simulink model "modele5Bhrolv2"  (R2024a)
settings: Solver=VariableStepAuto  StartTime=0.0  StopTime=100  RelTol=10e-2
undefined symbols (not defined in the file or in its folder): A_L, A_S, C_x, calcul_adherence, calcul_delta, calcul_forceaero, calcul_forces, calcul_lambda, calcul_moteur, calcul_N, calcul_omega, calcul_omegaackermann, calcul_retourvitesse, calcul_rotaroute, calcul_slipangle, calcul_vitessesroues, check_zeros_1, check_zeros_8, Cte_1, Cte_2, Cte_3, Cte_4, d_f, d_r, EPSILON, eqpfd, f, g, h, Iz, J, L, l_f, l_r, M, projection, R, reconstructionPi, rho
libraries: simulink x5, embmathops x1, slpidlib x1
settings Model: Creator=TP-EEA  LastModifiedBy=TP-EEA

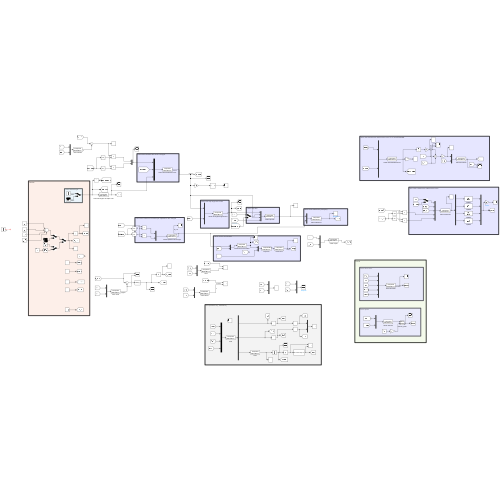
[thumbnail: Simulink's stored preview of the top-level diagram]
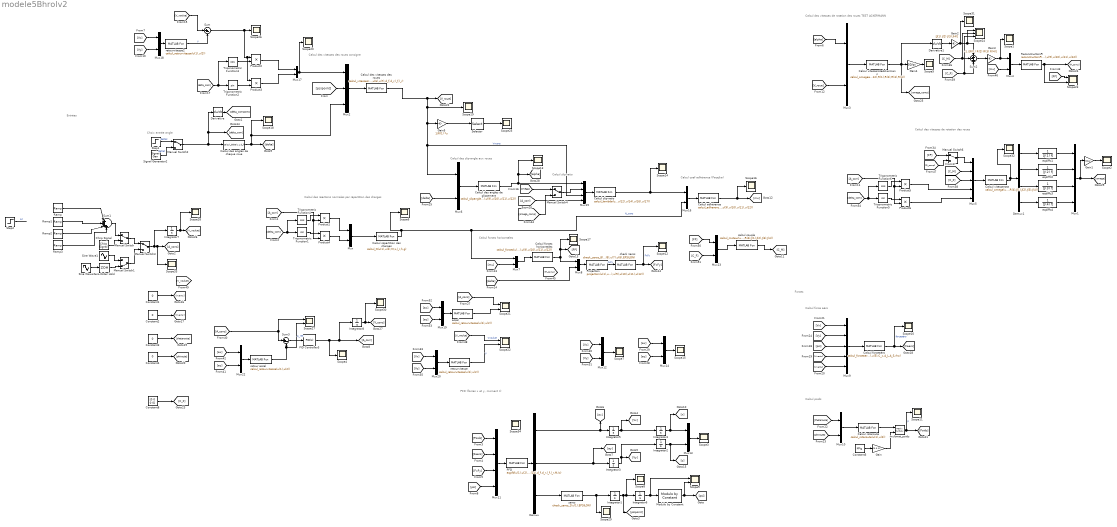
== system modele5Bhrolv2 ==
  note: Calcul des vitesses des roues consigne
  note: Entrées
  note: Choix entrée angle
  note: Calcul des vitesses de rotation des roues
  note: PFD (forces x et y, moment z)
  note: Calcul poids
  note: Calcul des slip-angle aux roues
  note: Calcul coef adhérence (Pacejka)
  note: Calcul slip-ratio
  note: Calcul des réactions normales par répartition des charges
  note: Calcul forces horizontales
  note: Forces
  note: Calcul force aéro
  note: Calcul des vitesses de rotation des roues TEST ACKERMANN
  Calcul adhérence : MATLABFcn  MATLABFcn=calcul_adherence(u(1),u(2),u(3),u(4),u(5),u(6),u(7),u(8),Cte_1,Cte_2,Cte_3,Cte_4,u(9),u(10),u(11),u(12))  OutputDimensions=4*2
  Calcul des angles de chaque roue : MATLABFcn  MATLABFcn=calcul_delta(u,L,d_f)  OutputDimensions=4
  Calcul des angles de glissement : MATLABFcn  MATLABFcn=calcul_slipangle(u(1),u(2),u(3),u(4),u(5),u(6),u(7),u(8),u(9),u(10),u(11),u(12))  OutputDimensions=4
  Calcul des vitesses des roues : MATLABFcn  MATLABFcn=calcul_vitessesroues(u(1),u(2),u(3),u(4),u(5),u(6),u(7),d_f,d_r,l_f,l_r)  OutputDimensions=8
  Calcul forceaéro : MATLABFcn  MATLABFcn=calcul_forceaero(u(1),u(2),u(3),u(4),u(5),C_x,A_L,A_S,rho)  OutputDimensions=2
  Calcul forces horizontales : MATLABFcn  MATLABFcn=calcul_forces(u(1),u(2),u(3),u(4),u(5),u(6),u(7),u(8),u(9),u(10),u(11),u(12))  OutputDimensions=4*2
  Calcul rotaroute : MATLABFcn  MATLABFcn=calcul_rotaroute(u(1),u(2))  OutputDimensions=[3 3]  Output1D=off
  Calcul répartition des charges : MATLABFcn  MATLABFcn=calcul_N(u(1),u(2),M,L,l_r,h,g)  OutputDimensions=4
  Calcul slip-ratio : MATLABFcn  MATLABFcn=calcul_lambda(u(1),u(2),u(3),u(4),R(1),R(2),R(3),R(4),u(5),u(6),u(7),u(8),u(9),u(11),u(13),u(15),u(10),u(12),u(14),u(16),u(17))  OutputDimensions=4*2
  Calcul vitesserota : MATLABFcn  MATLABFcn=calcul_omega(u(1),u(2),u(3),u(4),u(5),u(6),u(7),u(8),u(9),u(10),u(11),u(12),u(13),u(14),u(15),u(16),u(17),u(18),R(1),R(2),R(3),R(4),J(1),J(2),J(3),J(4))  OutputDimensions=4
  Calcul vitesserotaAckermann : MATLABFcn  MATLABFcn=calcul_omegaackermann(u(1),u(2),u(3),u(4),u(5),u(6),u(7),u(8),u(9),u(10),u(11),u(12),R(1),R(2),R(3),R(4))  OutputDimensions=4
  Chirp Signal : simulink/Sources/Chirp Signal  f1=0.1  T=100  f2=1
  Constant{1..4} (4 alike) : Constant  Value=0
  Constant5 : Constant  Value=M*g  VectorParams1D=off
  Constant8 : Constant  Value=[0 0 0 0]
  Demux : Demux  Outputs=3
  Demux1 : Demux
  Derivative : Derivative
  Derivative1 : Derivative
  Gain : Gain  Gain=[0 0 1]'
  Gain1 : Gain  Gain=30/pi
  Gain2 : Gain  Gain=[J(1) J(2) J(3) J(4)]
  Gain3 : Gain  Gain=-1./[R(1) R(2) R(3) R(4)]
  Gain4 : Gain  Gain=30/pi
  Gain5 : Gain  Gain=1/R(1)  Multiplication=Matrix(K*u)
  Integrator{1..8} (8 alike) : Integrator
  Manual Switch{,2..4,6} (5 alike) : ManualSwitch
  Manual Switch1 : ManualSwitch  CurrentSetting=0
  Modulo by Constant : embmathops/Modulo by Constant  Denominator=2*pi  SimulateUsing=Code generation
      settings: LibrarySourceBlock=embeddedMathLib/Modulo by Constant
  Mux{,3..4,6..8,10,12..14,16..20,22..23} (17 alike) : Mux  Inputs=2
  Mux1 : Mux
  Mux11 : Mux
  Mux15 : Mux
  Mux2 : Mux  Inputs=3
  Mux5 : Mux  Inputs=5
  Mux9 : Mux  Inputs=5
  PFD : MATLABFcn  MATLABFcn=eqpfd(u(1),u(2),u(4),u(5),u(6),u(7),u(8),u(9),u(10),u(11),u(12),u(13),u(14),d_f,d_r,l_f,l_r,M,Iz)  OutputDimensions=3
  PID Controller3 : slpidlib/PID Controller  Controller=PID  Form=Ideal  TimeDomain=Continuous-time  UseExternalTs=off  SampleTime=-1  IntegratorMethod=Forward Euler  FilterMethod=Forward Euler  ControllerParametersSource=internal  P=1  I=30  UseKiTs=off  D=0  UseExternalDerivativeSource=off  N=300  UseFilter=on  TunerSelectOption=Frequency Response Based  InitialConditionSource=internal  InitialConditionForIntegrator=0  InitialConditionForFilter=0  DifferentiatorICPrevScaledInput=0  ExternalReset=none  TrackingMode=off  Kt=1  LimitOutput=off  SatLimitsSource=internal  UpperSaturationLimit=inf  LowerSaturationLimit=-inf  LinearizeAsGain=on  AntiWindupMode=none  Kb=1  LimitIntegrator=off  UpperIntegratorSaturationLimit=inf  LowerIntegratorSaturationLimit=-inf  POutMin=[]  POutMax=[]  IOutMin=[]  IOutMax=[]  DOutMin=[]  DOutMax=[]  NOutMin=[]  NOutMax=[]  SumOutMin=[]  SumOutMax=[]  SaturationOutMin=[]  SaturationOutMax=[]  PParamMin=[]  PParamMax=[]  IParamMin=[]  IParamMax=[]  DParamMin=[]  DParamMax=[]  NParamMin=[]  NParamMax=[]  KbParamMin=[]  KbParamMax=[]  KtParamMin=[]  KtParamMax=[]  KbOutMin=[]  KbOutMax=[]  KtOutMin=[]  KtOutMax=[]  IntegratorOutMin=[]  IntegratorOutMax=[]  FilterOutMin=[]  FilterOutMax=[]  SumI1OutMin=[]  SumI1OutMax=[]  SumI2OutMin=[]  SumI2OutMax=[]  SumI3OutMin=[]  SumI3OutMax=[]  SumI4OutMin=[]  SumI4OutMax=[]  SumDOutMin=[]  SumDOutMax=[]  DifferentiatorOutMin=[]  DifferentiatorOutMax=[]  FilterDiffOutCoefMin=[]  FilterDiffOutCoefMax=[]  ReciprocalOutMin=[]  ReciprocalOutMax=[]  SumDenOutMin=[]  SumDenOutMax=[]  SumNumOutMin=[]  SumNumOutMax=[]  DivideOutMin=[]  DivideOutMax=[]  UdiffTsProdOutMin=[]  UdiffTsProdOutMax=[]  NTsProdOutMin=[]  NTsProdOutMax=[]  UintegralTsProdOutMin=[]  UintegralTsProdOutMax=[]  UngainTsProdOutMin=[]  UngainTsProdOutMax=[]  ClampingZeroOutDataTypeStr=Inherit: Inherit via back propagation  ClampingZeroOutMin=[]  ClampingZeroOutMax=[]  FilterDenConstantOutDataTypeStr=Inherit: Inherit via back propagation  FilterDenConstantOutMin=[]  FilterDenConstantOutMax=[]  PCopyOutDataTypeStr=Inherit: Inherit via back propagation  PCopyOutMin=[]  PCopyOutMax=[]  NCopyOutDataTypeStr=Inherit: Inherit via back propagation  NCopyOutMin=[]  NCopyOutMax=[]  IntegratorContinuousStateAttributes=''  IntegratorStateMustResolveToSignalObject=off  IntegratorRTWStateStorageClass=Auto  FilterContinuousStateAttributes=''  FilterStateMustResolveToSignalObject=off  FilterRTWStateStorageClass=Auto  ParallelPVariant=Passthrough  IdealPVariant=InternalParameters  IVariant=InternalParameters  DVariant=InternalParameters  IntegratorVariant=Continuous  SatVariant=Disabled  AWVariant=Passthrough  PCopyVariant=Disabled  TRVariant=Disabled  FdbkBlocksVariant=Forward  IdealPFdbkVariant=Disabled  SatFdbkVariant=Disabled  DerivativeFilterVariant=ContFilter  NVariant=InternalParameters  NCopyVariant=Disabled  FilterICVariant=InternalICsFilter  IntegratorICVariant=InternalICs  ExternalResetVariant=Disabled  TRSumVariant=Passthrough  SumFdbkVariant=Disabled  SumVariant=Sum_PID  TsampFilterVariant=InternalTs  TsampNgainVariant=Passthrough  TsampIntegralVariant=Disabled_SignalSpec  ExternalSaturationOutDataTypeStr=Inherit: Same as second input  DerivativeSourceVariant=ErrorSignal
  Product{1..6} (6 alike) : Product
  Projection : MATLABFcn  MATLABFcn=projection(u(1),u(2),u(3),u(4),u(5),u(6),u(7),u(8),u(9),u(10),u(11),u(12))  OutputDimensions=8
  Ramp : simulink/Sources/Ramp  slope=1  start=0  InitialOutput=0
  Ramp1 : simulink/Sources/Ramp  slope=-1  start=3  InitialOutput=0
  Ramp2 : simulink/Sources/Ramp  slope=-1  start=7  InitialOutput=0
  Ramp3 : simulink/Sources/Ramp  slope=1  start=9  InitialOutput=0
  ReconstructionPi : MATLABFcn  MATLABFcn=reconstructionPi(u(1),u(2),u(3),u(4),u(5),u(6),u(7),u(8),u(9),u(10),u(11),u(12))  OutputDimensions=8
  Scope{1..8,10..20,25..26,28..34} (28 alike) : Scope
  Scope{9,21..23,27} (5 alike) : Scope  NumInputPorts=2
  Scope24 : Scope  NumInputPorts=3
  Selector : Selector  InputPortWidth=8  IndexOptions=Index vector (dialog)  Indices=[1,3,5,7]  OutputSizes=1
  Signal Generator2 : SignalGenerator  Frequency=0.01  Units=rad/sec
  Sine Wave : Sin  SampleTime=0
  Sine Wave1 : Sin  SampleTime=0
  Step1 : Step  Time=0  After=0  SampleTime=0
  Step2 : Step  Time=3  After=3  SampleTime=0
  Sum : Sum  Inputs=|+-
  Sum1 : Sum  Inputs=|++++
  Sum2 : Sum  Inputs=+-+
  Sum3 : Sum  Inputs=|+-
  Trigonometric Function1 : Trigonometry
  Trigonometric Function2 : Trigonometry
  Trigonometric Function3 : Trigonometry  Operator=cos
  Trigonometric Function4 : Trigonometry  Operator=cos
  Trigonometric Function5 : Trigonometry
  Trigonometric Function6 : Trigonometry  Operator=cos
  Zero-Order Hold : ZeroOrderHold
  accel : MATLABFcn  MATLABFcn=calcul_retourvitesse(u(1),u(2))  OutputDimensions=1
  calcul couple : MATLABFcn  MATLABFcn=calcul_moteur(u(1),u(2),u(3),u(4),u(5),u(6),u(7),u(8),u(9),u(10),u(11),u(12),R(1),R(2),R(3),R(4),J(1),J(2),J(3),J(4))
  check zeros : MATLABFcn  MATLABFcn=check_zeros_8(u(1),u(2),u(3),u(4),u(5),u(6),u(7),u(8),EPSILON)  OutputDimensions=8
  eqdiffz1 : TransferFcn  Denominator=[J(1) f]
  eqdiffz2 : TransferFcn  Denominator=[J(2) f]
  eqdiffz3 : TransferFcn  Denominator=[J(3) f]
  eqdiffz4 : TransferFcn  Denominator=[J(4) f]
  multmat_poids : Product  Multiplication=Matrix(*)
  retour accel : MATLABFcn  MATLABFcn=calcul_retourvitesse(u(1),u(2))  OutputDimensions=1
  retourvitesse : MATLABFcn  MATLABFcn=calcul_retourvitesse(u(1),u(2))  OutputDimensions=1
  retourvitesse2 : MATLABFcn  MATLABFcn=calcul_retourvitesse(u(1),u(2))  OutputDimensions=1
  zeros : MATLABFcn  MATLABFcn=check_zeros_1(u(1),EPSILON)
  wires:
  accel/1 -> Scope21/2
  Calcul des angles de glissement/1 -> [alpha], Scope13/1, Mux15/1
  Mux17/1 -> Scope20/1, Mux2/1
  [Vventy] -> Mux9/5
  [ay] -> Mux22/2
  Mux16/1 -> Calcul adhérence/1
  [ax] -> Mux22/1
  Mux9/1 -> Calcul forceaéro/1
  Mux2/1 -> Calcul des vitesses des roues/1
  Calcul adhérence/1 -> [mu], Scope16/1
  [A_cons] -> Sum3/1, Scope27/1
  Mux22/1 -> retour accel/1
  [thetaroute] -> Mux10/1
  [Vx] -> Mux20/1
  eqdiffz4/1 -> Mux1/4
  [Faero] -> Mux11/2
  retourvitesse/1 -> Scope22/2  "V"
  Chirp Signal/1 -> Manual Switch/2
  [ax] -> Mux19/1
  Mux11/1 -> PFD/1
  [A_cons] -> Scope21/1
  [Poids] -> Mux11/1
  Manual Switch2/1 -> Derivative/1, [delta_com], Calcul des angles de chaque roue/1
  Trigonometric Function3/1 -> Product2/2
  Product2/1 -> Mux17/1
  Projection/1 -> check zeros/1  "FxFy"
  Trigonometric Function2/1 -> Product3/2
  [A_corr] -> Mux15/4
  PFD/1 -> Demux/1
  Mux8/1 -> Projection/1
  Constant5/1 -> Gain/1
  Mux6/1 -> Calcul des angles de glissement/1
  Integrator2/1 -> Mux13/2, [y]
  Mux7/1 -> Calcul forces horizontales/1
  multmat_poids/1 -> Scope11/1, [Poids]  "P"
  Product3/1 -> Mux17/2
  Mux10/1 -> Calcul rotaroute/1
  Calcul forceaéro/1 -> Scope10/1, [Faero]  "forceaéro"
  Integrator1/1 -> Scope8/1, Integrator6/1, [psipoint]
  Mux15/1 -> Calcul slip-ratio/1
  [FxFy] -> Mux11/3
  [delta_com] -> Trigonometric Function3/1, Trigonometric Function2/1
  Gain/1 -> multmat_poids/2
  Mux20/1 -> retourvitesse/1
  [mu] -> Mux7/2
  Mux14/1 -> Scope15/1
  [psipoint] -> Mux2/2
  Integrator4/1 -> Mux13/1, [x]
  [Vventx] -> Mux9/4
  [psi] -> Mux9/3
  [ax] -> Mux14/1
  [ay] -> Mux14/2
  Mux12/1 -> Scope7/1
  Integrator5/1 -> Integrator4/1, [Vx]
  [phiroute] -> Mux10/2
  Integrator6/1 -> Modulo by Constant/1, Scope9/1
  [Vx] -> Mux12/1
  Mux13/1 -> Scope3/1
  Signal Generator2/1 -> Manual Switch2/2  "delta*"
  eqdiffz3/1 -> Mux1/3
  calcul couple/1 -> [C_M]
  [Vy] -> Mux12/2
  Step1/1 -> Manual Switch2/1  "delta*"
  Calcul rotaroute/1 -> multmat_poids/1
  Constant1/1 -> [Vventx]
  Calcul des angles de chaque roue/1 -> [delta], Mux2/3, Scope18/1
  Derivative/1 -> [delta_compoint]
  Calcul répartition des charges/1 -> Mux16/2, Mux7/1, Scope6/1  "N_cons"
  [Vy] -> Mux9/2
  Constant4/1 -> [phiroute]
  Constant2/1 -> [Vventy]
  Integrator3/1 -> Integrator2/1, [Vy]
  Demux1/4 -> eqdiffz4/1
  Constant8/1 -> [C_F]
  eqdiffz2/1 -> Mux1/2
  [C_M] -> Mux5/2
  Mux19/1 -> accel/1
  Mux5/1 -> Calcul vitesserota/1
  Calcul vitesserota/1 -> Scope32/1, Demux1/1
  [delta] -> Mux8/2
  retour accel/1 -> Sum3/2, Scope27/2  "A_ret"
  Mux1/1 -> [omega], Gain1/1
  [C_F] -> Mux5/3
  eqdiffz1/1 -> Mux1/1
  Constant3/1 -> [thetaroute]
  Demux1/3 -> eqdiffz3/1
  Demux1/2 -> eqdiffz2/1
  Demux1/1 -> eqdiffz1/1
  Product4/1 -> Mux/2
  [A_corr] -> Product4/2, Product1/2
  [ay] -> Mux19/2
  [Vy] -> Mux20/2
  Modulo by Constant/1 -> [psi], Scope9/2
  Sine Wave/1 -> Zero-Order Hold/1
  Manual Switch3/1 -> Integrator7/1, Scope33/1, [A_cons]
  Manual Switch/1 -> Manual Switch3/1
  Manual Switch1/1 -> Manual Switch3/2
  Zero-Order Hold/1 -> Manual Switch1/2
  Sine Wave1/1 -> Manual Switch1/1
  Gain1/1 -> Scope2/1
  Step2/1 -> ?  "A*"
  Sum1/1 -> Manual Switch/1
  [V_roue] -> Mux3/2
  Mux3/1 -> Calcul vitesserotaAckermann/1
  Calcul vitesserotaAckermann/1 -> Gain4/1, Derivative1/1, [omega_comp]
  Derivative1/1 -> Gain2/1
  Gain2/1 -> Scope31/1, Scope24/1, Sum2/1
  [C_M] -> Scope24/2, Sum2/2
  [C_F] -> Scope24/3, Sum2/3
  Sum2/1 -> Gain3/1
  [FP] -> Scope23/1
  Manual Switch4/1 -> Mux15/2
  [omega_comp] -> Manual Switch4/2
  [mu] -> Mux4/2
  Gain3/1 -> Scope1/1, Mux4/1
  Mux4/1 -> ReconstructionPi/1
  ReconstructionPi/1 -> [Fi_comp], Scope23/2
  [FP] -> Manual Switch6/1
  Manual Switch6/1 -> Mux5/1
  [Fi_comp] -> Manual Switch6/2
  [V_voulue] -> Scope22/1  "Vvoulue"
  zeros/1 -> Scope29/1, Integrator1/1
  [Vx] -> Mux9/1
  Sum3/1 -> PID Controller3/1
  Gain4/1 -> Scope5/1
  Integrator8/1 -> Scope30/1, [V_cons]
  PID Controller3/1 -> Integrator8/1, [A_corr], Scope4/1
  Gain5/1 -> Selector/1
  Selector/1 -> Scope25/1
  [alpha] -> Mux3/1
  Demux/1 -> [ax], Integrator5/1
  Demux/2 -> [ay], Integrator3/1
  [Vy] -> Mux18/2
  [Vx] -> Mux18/1
  [V_voulue] -> Sum/1
  retourvitesse2/1 -> Sum/2  "V"
  Mux18/1 -> retourvitesse2/1
  [psi] -> Mux11/4
  [delta] -> Mux6/2
  [omega] -> Manual Switch4/1
  Product5/1 -> Mux5/4
  Product6/1 -> Mux5/5
  Calcul forces horizontales/1 -> Scope17/1, [FP], Mux8/1
  Calcul slip-ratio/1 -> Mux16/1, Scope14/1
  Mux/1 -> Calcul répartition des charges/1
  Calcul des vitesses des roues/1 -> Gain5/1, Mux6/1, Mux15/3, Scope19/1, [V_roue]  "Vrcons"
  Demux/3 -> zeros/1
  [FP] -> Mux23/1
  [C_F] -> Mux23/2
  Mux23/1 -> calcul couple/1
  check zeros/1 -> Scope12/1, [FxFy]  "FxFy"
  Sum/1 -> Scope26/1, Product3/1, Product2/1
  Ramp/1 -> Sum1/1
  Ramp1/1 -> Sum1/2
  Ramp2/1 -> Sum1/3
  Ramp3/1 -> Sum1/4
  Integrator7/1 -> [V_voulue], Scope28/1
  [delta_com] -> Trigonometric Function4/1, Trigonometric Function1/1
  Trigonometric Function1/1 -> Product4/1
  Trigonometric Function4/1 -> Product1/1
  Product1/1 -> Mux/1
  Trigonometric Function5/1 -> Product6/1
  Trigonometric Function6/1 -> Product5/1
  [A_corr] -> Product6/2, Product5/2
  [delta_com] -> Trigonometric Function6/1, Trigonometric Function5/1
